simulink model "Control"  (R2023b)
settings: Solver=ode4  StartTime=0.0  StopTime=13  FixedStep=0.001  RelTol=1e-3
undefined symbols (not defined in the file or in its folder): DiscIntNeverNeededParam
libraries: fl_lib x6, nesl_utility x4
settings Model: Creator=User  LastModifiedBy=User

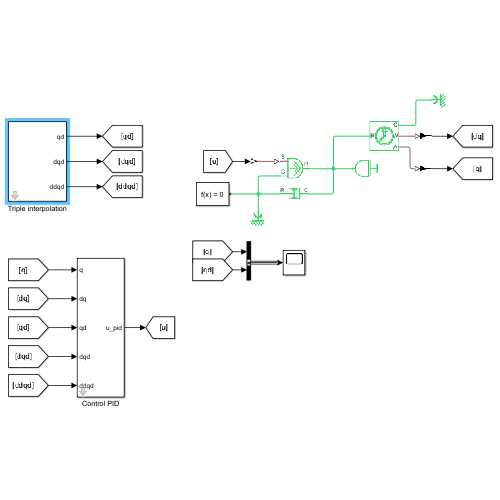
[thumbnail: Simulink's stored preview of the top-level diagram]
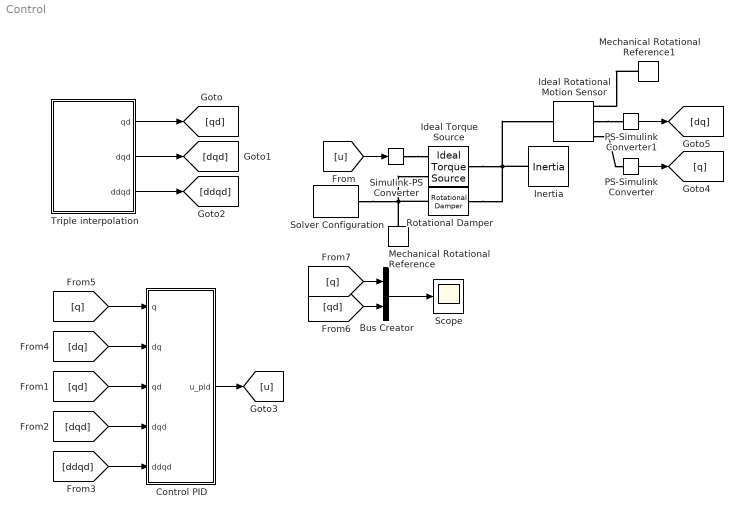
== system Control ==
  Bus Creator : BusCreator  Inputs=2
  Control PID : Subsystem  mask{J=768.8e-9, B=1.2, ts=0.1, Mp=110, ki=0.1}
      mask prompts: J "Inercia efectiva"; B "Amortiguamiento efectivo"; ts "Tiempo de establecimiento"; Mp "Maximo sobretiro"; ki "Ganancia Integral"
      mask init:
      | zeta = log(Mp/100)/sqrt(pi^2+(log(Mp/100))^2);
      | wn = 3/(zeta*ts);
      | PD = [1 2*zeta*wn wn^2];
      | kd = PD(2)-B/J;
      | kp = PD(3);
  Ideal Rotational Motion Sensor : fl_lib/Mechanical/Mechanical Sensors/Ideal Rotational Motion Sensor  reference=foundation.enum.MeasurementReference.difference  acceleration_port=false  velocity_port=true  position_port=true  wrap_angle=false  offset=0 rad
  Ideal Torque Source : fl_lib/Mechanical/Mechanical Sources/Ideal Torque Source
  Inertia : fl_lib/Mechanical/Rotational Elements/Inertia  inertia=768.8e-9 kg*m^2  num_ports=foundation.enum.numPorts2.one  w_specify=off  w_priority=High  w=0 rad/s  w_nominal_specify=off  w_nominal_unit=rad/s  w_nominal_value=1  t_specify=off  t_priority=None  t=0 N*m  t_nominal_specify=off  t_nominal_unit=N*m  t_nominal_value=1
  Mechanical Rotational Reference : fl_lib/Mechanical/Rotational Elements/Mechanical Rotational Reference
  Mechanical Rotational Reference1 : fl_lib/Mechanical/Rotational Elements/Mechanical Rotational Reference
  PS-Simulink Converter : nesl_utility/PS-Simulink Converter  PhysicalDomain=network_engine_domain  SubClassName=ps_output  LeftPortType=input  RightPortType=output  PseudoPeriodic=off  Frequencies=[]  VectorFormat=inherit  Unit=inherit  AffineConversion=off
  PS-Simulink Converter1 : nesl_utility/PS-Simulink Converter  PhysicalDomain=network_engine_domain  SubClassName=ps_output  LeftPortType=input  RightPortType=output  PseudoPeriodic=off  Frequencies=[]  VectorFormat=inherit  Unit=inherit  AffineConversion=off
  Rotational Damper : fl_lib/Mechanical/Rotational Elements/Rotational Damper  D=1.2 N*m*s/rad  w_specify=off  w_priority=None  w=0 rad/s  w_nominal_specify=off  w_nominal_unit=rad/s  w_nominal_value=1  t_specify=off  t_priority=None  t=0 N*m  t_nominal_specify=off  t_nominal_unit=N*m  t_nominal_value=1
  Scope : Scope
  Simulink-PS Converter : nesl_utility/Simulink-PS Converter  PhysicalDomain=network_engine_domain  SubClassName=ps_input  LeftPortType=input  RightPortType=output  PseudoPeriodic=off  Frequencies=[]  NoiseDistribution=none  NoiseParameters=[]  Unit=1  AffineConversion=off  FilteringAndDerivatives=provide  SimscapeFilterOrder=1  InputFilterTimeConstant=0.001  UdotUserProvided=0
  Solver Configuration : nesl_utility/Solver Configuration  PhysicalDomain=network_engine_domain  SubClassName=solver  LeftPortType=input  RightPortType=generic  Tones=[]  Harmonics=[]  SimulateNoise=off  Profile=off  UseLocalSampling=off  EnableSwitchedLinearOptims=on  FrequencyDomain=off  UseCCode=off  RelTol=0.001  AbsTol=0.001  MinStep=1e-09  ToWorkspace=off  RevertToSquareIcSolve=off  NumHomotopyIterations=100  PhasorMode=off  PhasorModeNumHarmonics=1  ConsistencySolver=NEWTON_XTOL_AFTER_FTOL  IndexReductionMethod=DerivativeReplacement  DoDC=off  ResidualTolerance=1e-09  ConsistencyTolSource=GLOBAL  ConsistencyAbsTol=0.001  ConsistencyRelTol=0.001  ConsistencyTolFactor=0.001  UseLocalSolver=off  LocalSolverChoice=NE_BACKWARD_EULER_ADVANCER  ResolveIndetEquations=on  FunctionEvalNumThread=1  LocalSolverSampleTime=0.001  DoFixedCost=off  MaxNonlinIter=3  MaxModeIter=2  ComputeImpulses=off  ImpulseIterations=2  LinearAlgebra=auto  LinearAlgebraNumThread=0  EquationFormulation=NE_TIME_EF  DelaysMemoryBudget=1024  AutomaticFiltering=on  FilteringTimeConstant=0.001  PartitionStorageMethod=AS_NEEDED  PartitionMemoryBudget=1024  PartitionMethod=ROBUST  MultibodyUseLocalSolver=off  MultibodyLocalSolverChoice=ODE1  MultibodyLocalSolverSampleTime=0.001
  Triple interpolation : Subsystem  mask{gain_trans=32, t_m=3, t_h=1}
      mask prompts: gain_trans "Transmission Gain"; t_m "Time of movement"; t_h "Time of hold"
  wires:
  PS-Simulink Converter/1 -> [q]
  PS-Simulink Converter1/1 -> [dq]
  [u] -> Simulink-PS Converter/1
  [qd] -> Control PID/3(qd)
  [dqd] -> Control PID/4(dqd)
  [ddqd] -> Control PID/5(ddqd)
  [dq] -> Control PID/2(dq)
  [q] -> Control PID/1(q)
  Control PID/1(u_pid) -> [u]
  [qd] -> Bus Creator/2
  Triple interpolation/1(qd) -> [qd]
  Triple interpolation/2(dqd) -> [dqd]
  Triple interpolation/3(ddqd) -> [ddqd]
  [q] -> Bus Creator/1
  Bus Creator/1 -> Scope/1
  connections:
  Simulink-PS Converter/RConn1 -- Ideal Torque Source/RConn1
  Mechanical Rotational Reference/LConn1 -- Rotational Damper/LConn1 -- Solver Configuration/RConn1 -- Ideal Torque Source/RConn2
  Ideal Torque Source/LConn1 -- Rotational Damper/RConn1 -- Ideal Rotational Motion Sensor/LConn1 -- Inertia/LConn1
  Mechanical Rotational Reference1/LConn1 -- Ideal Rotational Motion Sensor/RConn1
  Ideal Rotational Motion Sensor/RConn2 -- PS-Simulink Converter1/LConn1
  Ideal Rotational Motion Sensor/RConn3 -- PS-Simulink Converter/LConn1

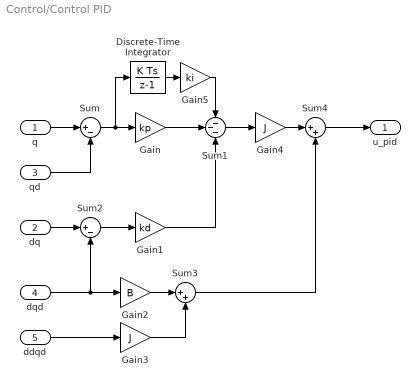
== system Control/Control PID ==
  q : Inport
  dq : Inport  Port=2
  qd : Inport  Port=3
  dqd : Inport  Port=4
  ddqd : Inport  Port=5
  Discrete-Time Integrator : DiscreteIntegrator  SampleTime=0.005  ICPrevOutput=DiscIntNeverNeededParam  ICPrevScaledInput=DiscIntNeverNeededParam
  Gain : Gain  Gain=kp
  Gain1 : Gain  Gain=kd
  Gain2 : Gain  Gain=B
  Gain3 : Gain  Gain=J
  Gain4 : Gain  Gain=J
  Gain5 : Gain  Gain=ki
  Sum : Sum  Inputs=|+-
  Sum1 : Sum  Inputs=---
  Sum2 : Sum  Inputs=|+-
  Sum3 : Sum  Inputs=|++
  Sum4 : Sum  Inputs=|++
  u_pid : Outport  VectorParamsAs1DForOutWhenUnconnected=off
  wires:
  dqd/1 -> Gain2/1, Sum2/2
  Gain2/1 -> Sum3/1
  dq/1 -> Sum2/1
  Sum1/1 -> Gain4/1
  Sum2/1 -> Gain1/1
  Sum4/1 -> u_pid/1
  ddqd/1 -> Gain3/1
  Sum/1 -> Discrete-Time Integrator/1, Gain/1
  q/1 -> Sum/1
  Gain4/1 -> Sum4/1
  Gain3/1 -> Sum3/2
  Sum3/1 -> Sum4/2
  qd/1 -> Sum/2
  Gain/1 -> Sum1/2
  Gain1/1 -> Sum1/3
  Gain5/1 -> Sum1/1
  Discrete-Time Integrator/1 -> Gain5/1

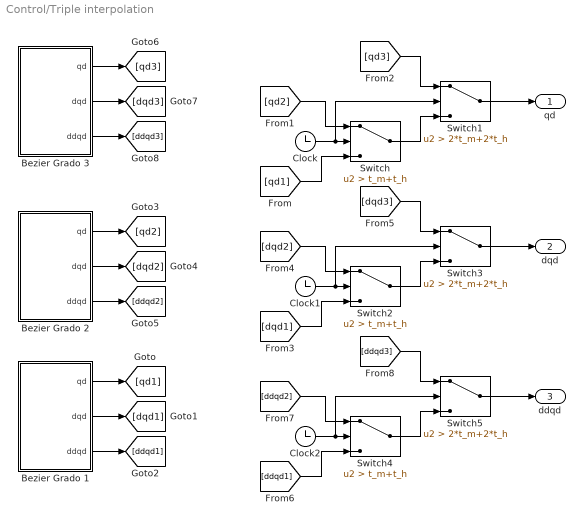
== system Control/Triple interpolation ==
  Bezier Grado 1 : Subsystem  mask{t1=t_h, t2=t_m+t_h, q1=0, q2=gain_trans*2*pi/3, gamma1=175.63, gamma2=548.18, gamma3=601.36, gamma4=216.36, gamma5=-45.81, gamma6=-34.36}
      mask prompts: t1 "Tiempo transicion 1"; t2 "Tiempo transicion 2"; q1 "Reposo inicial"; q2 "Reposo final"
  Bezier Grado 2 : Subsystem  mask{t1=t_m+2*t_h, t2=2*t_m+2*t_h, q1=gain_trans*2*pi/3, q2=gain_trans*4*pi/3, gamma1=175.63, gamma2=548.18, gamma3=601.36, gamma4=216.36, gamma5=-45.81, gamma6=-34.36}
      mask prompts: t1 "Tiempo transicion 1"; t2 "Tiempo transicion 2"; q1 "Reposo inicial"; q2 "Reposo final"
  Bezier Grado 3 : Subsystem  mask{t1=2*t_m+3*t_h, t2=3*t_m+3*t_h, q1=gain_trans*4*pi/3, q2=gain_trans*2*pi, gamma1=175.63, gamma2=548.18, gamma3=601.36, gamma4=216.36, gamma5=-45.81, gamma6=-34.36}
      mask prompts: t1 "Tiempo transicion 1"; t2 "Tiempo transicion 2"; q1 "Reposo inicial"; q2 "Reposo final"
  Clock : Clock
  Clock1 : Clock
  Clock2 : Clock
  Switch : Switch  Criteria=u2 > Threshold  Threshold=t_m+t_h  SaturateOnIntegerOverflow=off  InputSameDT=off
  Switch1 : Switch  Criteria=u2 > Threshold  Threshold=2*t_m+2*t_h  SaturateOnIntegerOverflow=off  InputSameDT=off
  Switch2 : Switch  Criteria=u2 > Threshold  Threshold=t_m+t_h  SaturateOnIntegerOverflow=off  InputSameDT=off
  Switch3 : Switch  Criteria=u2 > Threshold  Threshold=2*t_m+2*t_h  SaturateOnIntegerOverflow=off  InputSameDT=off
  Switch4 : Switch  Criteria=u2 > Threshold  Threshold=t_m+t_h  SaturateOnIntegerOverflow=off  InputSameDT=off
  Switch5 : Switch  Criteria=u2 > Threshold  Threshold=2*t_m+2*t_h  SaturateOnIntegerOverflow=off  InputSameDT=off
  qd : Outport
  dqd : Outport  Port=2
  ddqd : Outport  Port=3
  wires:
  Clock/1 -> Switch1/2, Switch/2
  Bezier Grado 1/1(qd) -> [qd1]
  Bezier Grado 1/2(dqd) -> [dqd1]
  Bezier Grado 1/3(ddqd) -> [ddqd1]
  Bezier Grado 2/1(qd) -> [qd2]
  Bezier Grado 2/2(dqd) -> [dqd2]
  Bezier Grado 2/3(ddqd) -> [ddqd2]
  Bezier Grado 3/1(qd) -> [qd3]
  Bezier Grado 3/2(dqd) -> [dqd3]
  Bezier Grado 3/3(ddqd) -> [ddqd3]
  [qd1] -> Switch/3
  [qd2] -> Switch/1
  Switch/1 -> Switch1/3
  [qd3] -> Switch1/1
  Switch1/1 -> qd/1
  [dqd3] -> Switch3/1
  Switch2/1 -> Switch3/3
  [dqd2] -> Switch2/1
  [dqd1] -> Switch2/3
  Clock1/1 -> Switch2/2, Switch3/2
  Switch3/1 -> dqd/1
  [ddqd3] -> Switch5/1
  Switch4/1 -> Switch5/3
  [ddqd2] -> Switch4/1
  Clock2/1 -> Switch5/2, Switch4/2
  [ddqd1] -> Switch4/3
  Switch5/1 -> ddqd/1

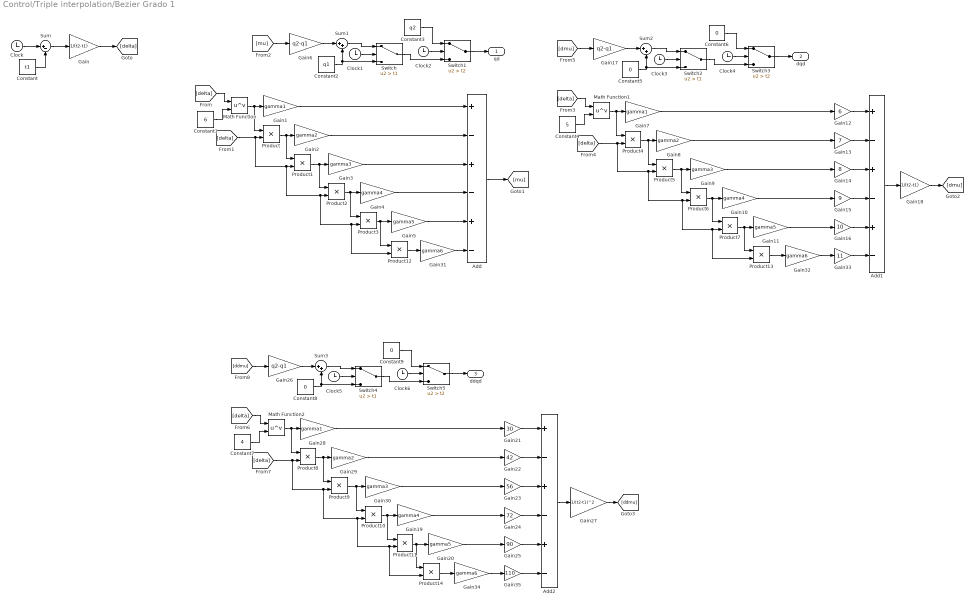
== system Control/Triple interpolation/Bezier Grado 1 ==
  Add : Sum  Inputs=+-+-+-
  Add1 : Sum  Inputs=+-+-+-
  Add2 : Sum  Inputs=+-+-+-
  Clock{,1..6} (7 alike) : Clock
  Constant : Constant  Value=t1
  Constant1 : Constant  Value=6
  Constant2 : Constant  Value=q1
  Constant3 : Constant  Value=q2
  Constant4 : Constant  Value=5
  Constant{5..6,8..9} (4 alike) : Constant  Value=0
  Constant7 : Constant  Value=4
  Gain : Gain  Gain=1/(t2-t1)
  Gain1 : Gain  Gain=gamma1
  Gain10 : Gain  Gain=gamma4
  Gain11 : Gain  Gain=gamma5
  Gain12 : Gain  Gain=6
  Gain13 : Gain  Gain=7
  Gain14 : Gain  Gain=8
  Gain15 : Gain  Gain=9
  Gain16 : Gain  Gain=10
  Gain17 : Gain  Gain=q2-q1
  Gain18 : Gain  Gain=1/(t2-t1)
  Gain19 : Gain  Gain=gamma4
  Gain2 : Gain  Gain=gamma2
  Gain20 : Gain  Gain=gamma5
  Gain21 : Gain  Gain=30
  Gain22 : Gain  Gain=42
  Gain23 : Gain  Gain=56
  Gain24 : Gain  Gain=72
  Gain25 : Gain  Gain=90
  Gain26 : Gain  Gain=q2-q1
  Gain27 : Gain  Gain=1/(t2-t1)^2
  Gain28 : Gain  Gain=gamma1
  Gain29 : Gain  Gain=gamma2
  Gain3 : Gain  Gain=gamma3
  Gain30 : Gain  Gain=gamma3
  Gain31 : Gain  Gain=gamma6
  Gain32 : Gain  Gain=gamma6
  Gain33 : Gain  Gain=11
  Gain34 : Gain  Gain=gamma6
  Gain35 : Gain  Gain=110
  Gain4 : Gain  Gain=gamma4
  Gain5 : Gain  Gain=gamma5
  Gain6 : Gain  Gain=q2-q1
  Gain7 : Gain  Gain=gamma1
  Gain8 : Gain  Gain=gamma2
  Gain9 : Gain  Gain=gamma3
  Math Function : Math  Operator=pow  SignedPower=on
  Math Function1 : Math  Operator=pow  SignedPower=on
  Math Function2 : Math  Operator=pow  SignedPower=on
  Product{,1..14} (15 alike) : Product
  Sum : Sum  Inputs=|+-
  Sum1 : Sum  Inputs=|++
  Sum2 : Sum  Inputs=|++
  Sum3 : Sum  Inputs=|++
  Switch : Switch  Criteria=u2 > Threshold  Threshold=t1  SaturateOnIntegerOverflow=off  InputSameDT=off
  Switch1 : Switch  Criteria=u2 > Threshold  Threshold=t2  SaturateOnIntegerOverflow=off  InputSameDT=off
  Switch2 : Switch  Criteria=u2 > Threshold  Threshold=t1  SaturateOnIntegerOverflow=off  InputSameDT=off
  Switch3 : Switch  Criteria=u2 > Threshold  Threshold=t2  SaturateOnIntegerOverflow=off  InputSameDT=off
  Switch4 : Switch  Criteria=u2 > Threshold  Threshold=t1  SaturateOnIntegerOverflow=off  InputSameDT=off
  Switch5 : Switch  Criteria=u2 > Threshold  Threshold=t2  SaturateOnIntegerOverflow=off  InputSameDT=off
  qd : Outport  VectorParamsAs1DForOutWhenUnconnected=off
  dqd : Outport  Port=2  VectorParamsAs1DForOutWhenUnconnected=off
  ddqd : Outport  Port=3  VectorParamsAs1DForOutWhenUnconnected=off
  wires:
  Gain35/1 -> Add2/6
  Gain34/1 -> Gain35/1
  Product14/1 -> Gain34/1
  Gain33/1 -> Add1/6
  Product13/1 -> Gain32/1
  Gain32/1 -> Gain33/1
  Gain31/1 -> Add/6
  Product12/1 -> Gain31/1
  [delta] -> Math Function2/1
  Product8/1 -> Gain29/1, Product9/1
  Constant7/1 -> Math Function2/2
  Product11/1 -> Product14/1, Gain20/1
  Product9/1 -> Gain30/1, Product10/1
  Product10/1 -> Gain19/1, Product11/1
  Math Function2/1 -> Gain28/1, Product8/1
  [delta] -> Product8/2, Product9/2, Product10/2, Product11/2, Product14/2
  Gain21/1 -> Add2/1
  Gain22/1 -> Add2/2
  Gain23/1 -> Add2/3
  Gain24/1 -> Add2/4
  Gain25/1 -> Add2/5
  Gain29/1 -> Gain22/1
  Gain28/1 -> Gain21/1
  Gain30/1 -> Gain23/1
  Gain19/1 -> Gain24/1
  Gain20/1 -> Gain25/1
  Switch4/1 -> Switch5/3
  Switch5/1 -> ddqd/1
  Gain26/1 -> Sum3/1
  Clock6/1 -> Switch5/2
  Clock5/1 -> Switch4/2
  Constant9/1 -> Switch5/1
  Sum3/1 -> Switch4/1
  [ddmu] -> Gain26/1
  Constant8/1 -> Sum3/2, Switch4/3
  Add2/1 -> Gain27/1
  Gain27/1 -> [ddmu]
  Gain18/1 -> [dmu]
  Add1/1 -> Gain18/1
  Constant5/1 -> Switch2/3, Sum2/2
  [dmu] -> Gain17/1
  Sum2/1 -> Switch2/1
  Constant6/1 -> Switch3/1
  Clock3/1 -> Switch2/2
  Clock4/1 -> Switch3/2
  Gain17/1 -> Sum2/1
  Switch3/1 -> dqd/1
  Switch2/1 -> Switch3/3
  Gain11/1 -> Gain16/1
  Gain10/1 -> Gain15/1
  Gain9/1 -> Gain14/1
  Gain7/1 -> Gain12/1
  Gain8/1 -> Gain13/1
  Gain16/1 -> Add1/5
  Gain15/1 -> Add1/4
  Gain14/1 -> Add1/3
  Gain13/1 -> Add1/2
  Gain12/1 -> Add1/1
  [delta] -> Product7/2, Product13/2, Product6/2, Product5/2, Product4/2
  Math Function1/1 -> Product4/1, Gain7/1
  Product6/1 -> Product7/1, Gain10/1
  Product5/1 -> Product6/1, Gain9/1
  Product7/1 -> Gain11/1, Product13/1
  Constant4/1 -> Math Function1/2
  Product4/1 -> Product5/1, Gain8/1
  [delta] -> Math Function1/1
  Switch/1 -> Switch1/3
  Switch1/1 -> qd/1
  Gain6/1 -> Sum1/1
  Gain2/1 -> Add/2
  [delta] -> Math Function/1
  Gain4/1 -> Add/4
  Gain/1 -> [delta]
  Gain3/1 -> Add/3
  Product/1 -> Gain2/1, Product1/1
  Clock2/1 -> Switch1/2
  Gain1/1 -> Add/1
  Clock1/1 -> Switch/2
  Constant1/1 -> Math Function/2
  Product3/1 -> Gain5/1, Product12/1
  Constant3/1 -> Switch1/1
  Product1/1 -> Gain3/1, Product2/1
  Add/1 -> [mu]
  Product2/1 -> Gain4/1, Product3/1
  Math Function/1 -> Gain1/1, Product/1
  Clock/1 -> Sum/1
  Sum1/1 -> Switch/1
  [mu] -> Gain6/1
  Sum/1 -> Gain/1
  Constant2/1 -> Sum1/2, Switch/3
  Gain5/1 -> Add/5
  Constant/1 -> Sum/2
  [delta] -> Product/2, Product1/2, Product2/2, Product3/2, Product12/2

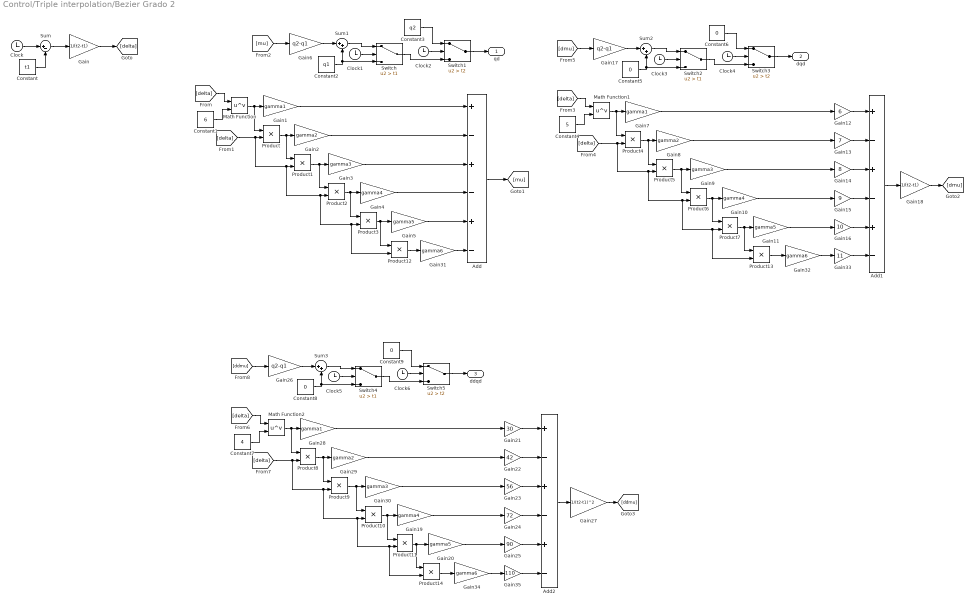
== system Control/Triple interpolation/Bezier Grado 2 ==
  Add : Sum  Inputs=+-+-+-
  Add1 : Sum  Inputs=+-+-+-
  Add2 : Sum  Inputs=+-+-+-
  Clock{,1..6} (7 alike) : Clock
  Constant : Constant  Value=t1
  Constant1 : Constant  Value=6
  Constant2 : Constant  Value=q1
  Constant3 : Constant  Value=q2
  Constant4 : Constant  Value=5
  Constant{5..6,8..9} (4 alike) : Constant  Value=0
  Constant7 : Constant  Value=4
  Gain : Gain  Gain=1/(t2-t1)
  Gain1 : Gain  Gain=gamma1
  Gain10 : Gain  Gain=gamma4
  Gain11 : Gain  Gain=gamma5
  Gain12 : Gain  Gain=6
  Gain13 : Gain  Gain=7
  Gain14 : Gain  Gain=8
  Gain15 : Gain  Gain=9
  Gain16 : Gain  Gain=10
  Gain17 : Gain  Gain=q2-q1
  Gain18 : Gain  Gain=1/(t2-t1)
  Gain19 : Gain  Gain=gamma4
  Gain2 : Gain  Gain=gamma2
  Gain20 : Gain  Gain=gamma5
  Gain21 : Gain  Gain=30
  Gain22 : Gain  Gain=42
  Gain23 : Gain  Gain=56
  Gain24 : Gain  Gain=72
  Gain25 : Gain  Gain=90
  Gain26 : Gain  Gain=q2-q1
  Gain27 : Gain  Gain=1/(t2-t1)^2
  Gain28 : Gain  Gain=gamma1
  Gain29 : Gain  Gain=gamma2
  Gain3 : Gain  Gain=gamma3
  Gain30 : Gain  Gain=gamma3
  Gain31 : Gain  Gain=gamma6
  Gain32 : Gain  Gain=gamma6
  Gain33 : Gain  Gain=11
  Gain34 : Gain  Gain=gamma6
  Gain35 : Gain  Gain=110
  Gain4 : Gain  Gain=gamma4
  Gain5 : Gain  Gain=gamma5
  Gain6 : Gain  Gain=q2-q1
  Gain7 : Gain  Gain=gamma1
  Gain8 : Gain  Gain=gamma2
  Gain9 : Gain  Gain=gamma3
  Math Function : Math  Operator=pow  SignedPower=on
  Math Function1 : Math  Operator=pow  SignedPower=on
  Math Function2 : Math  Operator=pow  SignedPower=on
  Product{,1..14} (15 alike) : Product
  Sum : Sum  Inputs=|+-
  Sum1 : Sum  Inputs=|++
  Sum2 : Sum  Inputs=|++
  Sum3 : Sum  Inputs=|++
  Switch : Switch  Criteria=u2 > Threshold  Threshold=t1  SaturateOnIntegerOverflow=off  InputSameDT=off
  Switch1 : Switch  Criteria=u2 > Threshold  Threshold=t2  SaturateOnIntegerOverflow=off  InputSameDT=off
  Switch2 : Switch  Criteria=u2 > Threshold  Threshold=t1  SaturateOnIntegerOverflow=off  InputSameDT=off
  Switch3 : Switch  Criteria=u2 > Threshold  Threshold=t2  SaturateOnIntegerOverflow=off  InputSameDT=off
  Switch4 : Switch  Criteria=u2 > Threshold  Threshold=t1  SaturateOnIntegerOverflow=off  InputSameDT=off
  Switch5 : Switch  Criteria=u2 > Threshold  Threshold=t2  SaturateOnIntegerOverflow=off  InputSameDT=off
  qd : Outport  VectorParamsAs1DForOutWhenUnconnected=off
  dqd : Outport  Port=2  VectorParamsAs1DForOutWhenUnconnected=off
  ddqd : Outport  Port=3  VectorParamsAs1DForOutWhenUnconnected=off
  wires:
  [delta] -> Product12/2, Product3/2, Product2/2, Product1/2, Product/2
  Constant/1 -> Sum/2
  Gain5/1 -> Add/5
  Constant2/1 -> Switch/3, Sum1/2
  Sum/1 -> Gain/1
  [mu] -> Gain6/1
  Sum1/1 -> Switch/1
  Clock/1 -> Sum/1
  Math Function/1 -> Product/1, Gain1/1
  Product2/1 -> Product3/1, Gain4/1
  Add/1 -> [mu]
  Product1/1 -> Product2/1, Gain3/1
  Constant3/1 -> Switch1/1
  Product3/1 -> Product12/1, Gain5/1
  Constant1/1 -> Math Function/2
  Clock1/1 -> Switch/2
  Gain1/1 -> Add/1
  Clock2/1 -> Switch1/2
  Product/1 -> Product1/1, Gain2/1
  Gain3/1 -> Add/3
  Gain/1 -> [delta]
  Gain4/1 -> Add/4
  [delta] -> Math Function/1
  Gain2/1 -> Add/2
  Gain6/1 -> Sum1/1
  Switch1/1 -> qd/1
  Switch/1 -> Switch1/3
  [delta] -> Math Function1/1
  Product4/1 -> Gain8/1, Product5/1
  Constant4/1 -> Math Function1/2
  Product7/1 -> Product13/1, Gain11/1
  Product5/1 -> Gain9/1, Product6/1
  Product6/1 -> Gain10/1, Product7/1
  Math Function1/1 -> Gain7/1, Product4/1
  [delta] -> Product4/2, Product5/2, Product6/2, Product13/2, Product7/2
  Gain12/1 -> Add1/1
  Gain13/1 -> Add1/2
  Gain14/1 -> Add1/3
  Gain15/1 -> Add1/4
  Gain16/1 -> Add1/5
  Gain8/1 -> Gain13/1
  Gain7/1 -> Gain12/1
  Gain9/1 -> Gain14/1
  Gain10/1 -> Gain15/1
  Gain11/1 -> Gain16/1
  Switch2/1 -> Switch3/3
  Switch3/1 -> dqd/1
  Gain17/1 -> Sum2/1
  Clock4/1 -> Switch3/2
  Clock3/1 -> Switch2/2
  Constant6/1 -> Switch3/1
  Sum2/1 -> Switch2/1
  [dmu] -> Gain17/1
  Constant5/1 -> Sum2/2, Switch2/3
  Add1/1 -> Gain18/1
  Gain18/1 -> [dmu]
  Gain27/1 -> [ddmu]
  Add2/1 -> Gain27/1
  Constant8/1 -> Switch4/3, Sum3/2
  [ddmu] -> Gain26/1
  Sum3/1 -> Switch4/1
  Constant9/1 -> Switch5/1
  Clock5/1 -> Switch4/2
  Clock6/1 -> Switch5/2
  Gain26/1 -> Sum3/1
  Switch5/1 -> ddqd/1
  Switch4/1 -> Switch5/3
  Gain20/1 -> Gain25/1
  Gain19/1 -> Gain24/1
  Gain30/1 -> Gain23/1
  Gain28/1 -> Gain21/1
  Gain29/1 -> Gain22/1
  Gain25/1 -> Add2/5
  Gain24/1 -> Add2/4
  Gain23/1 -> Add2/3
  Gain22/1 -> Add2/2
  Gain21/1 -> Add2/1
  [delta] -> Product14/2, Product11/2, Product10/2, Product9/2, Product8/2
  Math Function2/1 -> Product8/1, Gain28/1
  Product10/1 -> Product11/1, Gain19/1
  Product9/1 -> Product10/1, Gain30/1
  Product11/1 -> Gain20/1, Product14/1
  Constant7/1 -> Math Function2/2
  Product8/1 -> Product9/1, Gain29/1
  [delta] -> Math Function2/1
  Product12/1 -> Gain31/1
  Gain31/1 -> Add/6
  Gain32/1 -> Gain33/1
  Product13/1 -> Gain32/1
  Gain33/1 -> Add1/6
  Product14/1 -> Gain34/1
  Gain34/1 -> Gain35/1
  Gain35/1 -> Add2/6

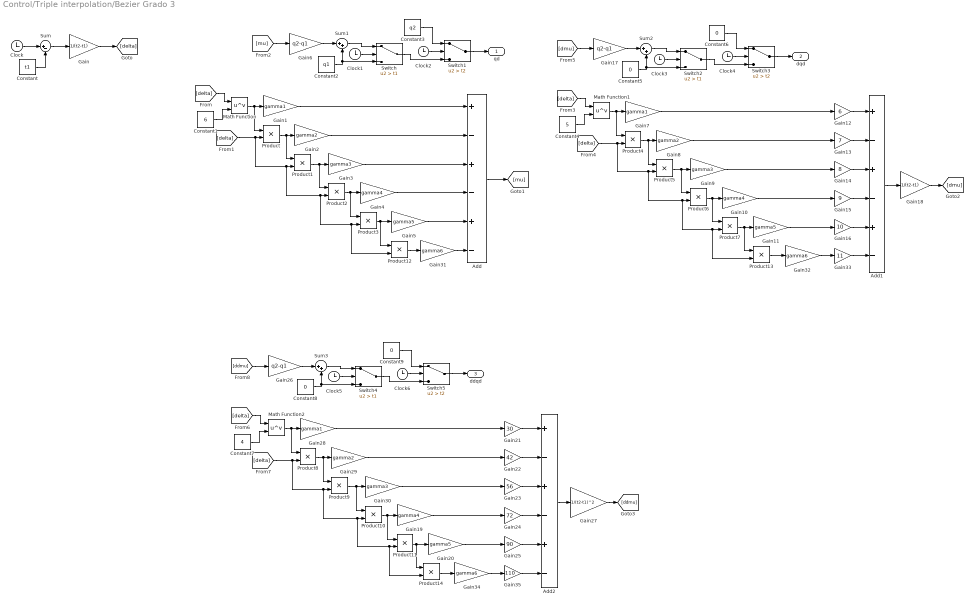
== system Control/Triple interpolation/Bezier Grado 3 ==
  Add : Sum  Inputs=+-+-+-
  Add1 : Sum  Inputs=+-+-+-
  Add2 : Sum  Inputs=+-+-+-
  Clock{,1..6} (7 alike) : Clock
  Constant : Constant  Value=t1
  Constant1 : Constant  Value=6
  Constant2 : Constant  Value=q1
  Constant3 : Constant  Value=q2
  Constant4 : Constant  Value=5
  Constant{5..6,8..9} (4 alike) : Constant  Value=0
  Constant7 : Constant  Value=4
  Gain : Gain  Gain=1/(t2-t1)
  Gain1 : Gain  Gain=gamma1
  Gain10 : Gain  Gain=gamma4
  Gain11 : Gain  Gain=gamma5
  Gain12 : Gain  Gain=6
  Gain13 : Gain  Gain=7
  Gain14 : Gain  Gain=8
  Gain15 : Gain  Gain=9
  Gain16 : Gain  Gain=10
  Gain17 : Gain  Gain=q2-q1
  Gain18 : Gain  Gain=1/(t2-t1)
  Gain19 : Gain  Gain=gamma4
  Gain2 : Gain  Gain=gamma2
  Gain20 : Gain  Gain=gamma5
  Gain21 : Gain  Gain=30
  Gain22 : Gain  Gain=42
  Gain23 : Gain  Gain=56
  Gain24 : Gain  Gain=72
  Gain25 : Gain  Gain=90
  Gain26 : Gain  Gain=q2-q1
  Gain27 : Gain  Gain=1/(t2-t1)^2
  Gain28 : Gain  Gain=gamma1
  Gain29 : Gain  Gain=gamma2
  Gain3 : Gain  Gain=gamma3
  Gain30 : Gain  Gain=gamma3
  Gain31 : Gain  Gain=gamma6
  Gain32 : Gain  Gain=gamma6
  Gain33 : Gain  Gain=11
  Gain34 : Gain  Gain=gamma6
  Gain35 : Gain  Gain=110
  Gain4 : Gain  Gain=gamma4
  Gain5 : Gain  Gain=gamma5
  Gain6 : Gain  Gain=q2-q1
  Gain7 : Gain  Gain=gamma1
  Gain8 : Gain  Gain=gamma2
  Gain9 : Gain  Gain=gamma3
  Math Function : Math  Operator=pow  SignedPower=on
  Math Function1 : Math  Operator=pow  SignedPower=on
  Math Function2 : Math  Operator=pow  SignedPower=on
  Product{,1..14} (15 alike) : Product
  Sum : Sum  Inputs=|+-
  Sum1 : Sum  Inputs=|++
  Sum2 : Sum  Inputs=|++
  Sum3 : Sum  Inputs=|++
  Switch : Switch  Criteria=u2 > Threshold  Threshold=t1  SaturateOnIntegerOverflow=off  InputSameDT=off
  Switch1 : Switch  Criteria=u2 > Threshold  Threshold=t2  SaturateOnIntegerOverflow=off  InputSameDT=off
  Switch2 : Switch  Criteria=u2 > Threshold  Threshold=t1  SaturateOnIntegerOverflow=off  InputSameDT=off
  Switch3 : Switch  Criteria=u2 > Threshold  Threshold=t2  SaturateOnIntegerOverflow=off  InputSameDT=off
  Switch4 : Switch  Criteria=u2 > Threshold  Threshold=t1  SaturateOnIntegerOverflow=off  InputSameDT=off
  Switch5 : Switch  Criteria=u2 > Threshold  Threshold=t2  SaturateOnIntegerOverflow=off  InputSameDT=off
  qd : Outport  VectorParamsAs1DForOutWhenUnconnected=off
  dqd : Outport  Port=2  VectorParamsAs1DForOutWhenUnconnected=off
  ddqd : Outport  Port=3  VectorParamsAs1DForOutWhenUnconnected=off
  wires:
  [delta] -> Product12/2, Product3/2, Product2/2, Product1/2, Product/2
  Constant/1 -> Sum/2
  Gain5/1 -> Add/5
  Constant2/1 -> Switch/3, Sum1/2
  Sum/1 -> Gain/1
  [mu] -> Gain6/1
  Sum1/1 -> Switch/1
  Clock/1 -> Sum/1
  Math Function/1 -> Product/1, Gain1/1
  Product2/1 -> Product3/1, Gain4/1
  Add/1 -> [mu]
  Product1/1 -> Product2/1, Gain3/1
  Constant3/1 -> Switch1/1
  Product3/1 -> Product12/1, Gain5/1
  Constant1/1 -> Math Function/2
  Clock1/1 -> Switch/2
  Gain1/1 -> Add/1
  Clock2/1 -> Switch1/2
  Product/1 -> Product1/1, Gain2/1
  Gain3/1 -> Add/3
  Gain/1 -> [delta]
  Gain4/1 -> Add/4
  [delta] -> Math Function/1
  Gain2/1 -> Add/2
  Gain6/1 -> Sum1/1
  Switch1/1 -> qd/1
  Switch/1 -> Switch1/3
  [delta] -> Math Function1/1
  Product4/1 -> Gain8/1, Product5/1
  Constant4/1 -> Math Function1/2
  Product7/1 -> Product13/1, Gain11/1
  Product5/1 -> Gain9/1, Product6/1
  Product6/1 -> Gain10/1, Product7/1
  Math Function1/1 -> Gain7/1, Product4/1
  [delta] -> Product4/2, Product5/2, Product6/2, Product13/2, Product7/2
  Gain12/1 -> Add1/1
  Gain13/1 -> Add1/2
  Gain14/1 -> Add1/3
  Gain15/1 -> Add1/4
  Gain16/1 -> Add1/5
  Gain8/1 -> Gain13/1
  Gain7/1 -> Gain12/1
  Gain9/1 -> Gain14/1
  Gain10/1 -> Gain15/1
  Gain11/1 -> Gain16/1
  Switch2/1 -> Switch3/3
  Switch3/1 -> dqd/1
  Gain17/1 -> Sum2/1
  Clock4/1 -> Switch3/2
  Clock3/1 -> Switch2/2
  Constant6/1 -> Switch3/1
  Sum2/1 -> Switch2/1
  [dmu] -> Gain17/1
  Constant5/1 -> Sum2/2, Switch2/3
  Add1/1 -> Gain18/1
  Gain18/1 -> [dmu]
  Gain27/1 -> [ddmu]
  Add2/1 -> Gain27/1
  Constant8/1 -> Switch4/3, Sum3/2
  [ddmu] -> Gain26/1
  Sum3/1 -> Switch4/1
  Constant9/1 -> Switch5/1
  Clock5/1 -> Switch4/2
  Clock6/1 -> Switch5/2
  Gain26/1 -> Sum3/1
  Switch5/1 -> ddqd/1
  Switch4/1 -> Switch5/3
  Gain20/1 -> Gain25/1
  Gain19/1 -> Gain24/1
  Gain30/1 -> Gain23/1
  Gain28/1 -> Gain21/1
  Gain29/1 -> Gain22/1
  Gain25/1 -> Add2/5
  Gain24/1 -> Add2/4
  Gain23/1 -> Add2/3
  Gain22/1 -> Add2/2
  Gain21/1 -> Add2/1
  [delta] -> Product14/2, Product11/2, Product10/2, Product9/2, Product8/2
  Math Function2/1 -> Product8/1, Gain28/1
  Product10/1 -> Product11/1, Gain19/1
  Product9/1 -> Product10/1, Gain30/1
  Product11/1 -> Gain20/1, Product14/1
  Constant7/1 -> Math Function2/2
  Product8/1 -> Product9/1, Gain29/1
  [delta] -> Math Function2/1
  Product12/1 -> Gain31/1
  Gain31/1 -> Add/6
  Gain32/1 -> Gain33/1
  Product13/1 -> Gain32/1
  Gain33/1 -> Add1/6
  Product14/1 -> Gain34/1
  Gain34/1 -> Gain35/1
  Gain35/1 -> Add2/6
